simulink subsystem "AAI"  (R2022a)
settings: Solver=VariableStepAuto  StartTime=0.0  StopTime=10.0  RelTol=1e-3
settings Model: Creator=bkfre  LastModifiedBy=bkfre

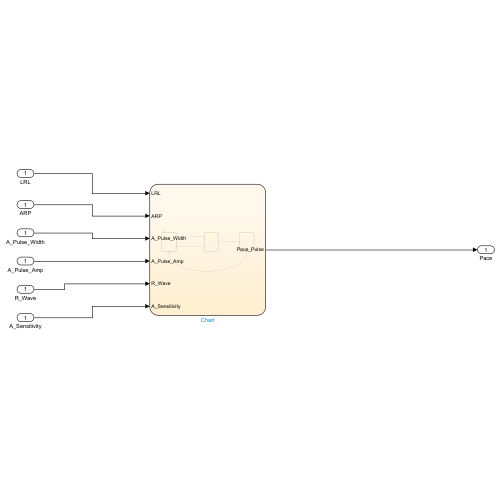
[thumbnail: Simulink's stored preview of the top-level diagram]
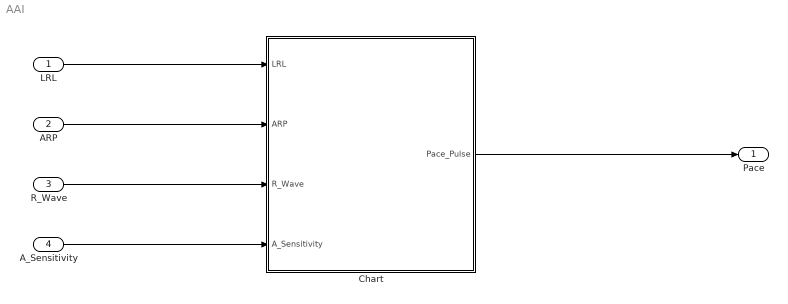
== system AAI ==
  LRL : Inport
  ARP : Inport  Port=2
  R_Wave : Inport  Port=3
  A_Sensitivity : Inport  Port=4
  Chart : Stateflow chart  TreatAsAtomicUnit=on
  Pace : Outport
  wires:
  R_Wave/1 -> Chart/3(R_Wave)
  Chart/1(Pace_Pulse) -> Pace/1
  A_Sensitivity/1 -> Chart/4(A_Sensitivity)
  ARP/1 -> Chart/2(ARP)
  LRL/1 -> Chart/1(LRL)

== stateflow chart AAI/Chart ==
  state Refractory
    entry:
    Pace_Pulse=0;
  state Alert
  state Pace
    entry:
    Pace_Pulse=1;
  (default) -> Refractory
  Refractory -> Alert : after(ARP,msec)
  Alert -> Pace [order 2] : after(LRL-ARP,msec)
  Alert -> Refractory [order 1] : [R_Wave>A_Sensitivity]
  Pace -> Refractory
  data: LRL input; ARP input; R_Wave input; Pace_Pulse output; A_Sensitivity input
